simulink model "Modelling"  (R2024b)
settings: Solver=ode15s  StartTime=0.0  StopTime=3*T0  RelTol=1e-7  AbsTol=1e-7
values from neighbouring files (symbols this model uses):
  omega0 = 0    [Numerical_model_1.m]    (also in Numerical_model_2.m = params.omega0)
  omegas = params.omegas    [Numerical_model_2.m]
undefined symbols (not defined in the file or in its folder): params
libraries: fl_lib x26, nesl_utility x12, ee_lib x1
settings Model: Creator=Mihnea  LastModifiedBy=Mihnea
settings SolverCC: AutoScaleAbsTol=off  SolverResetMethod=Robust
settings SimscapeCC: SimscapeLogType=all

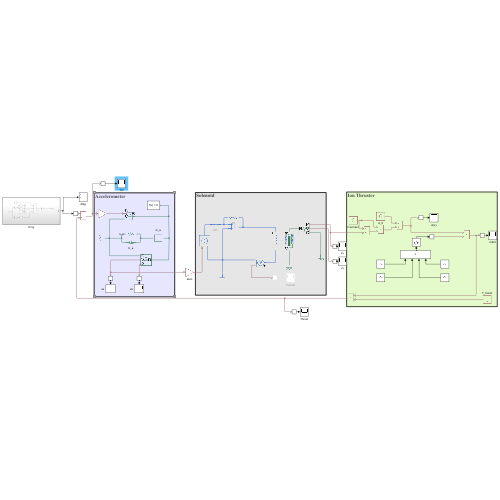
[thumbnail: Simulink's stored preview of the top-level diagram]
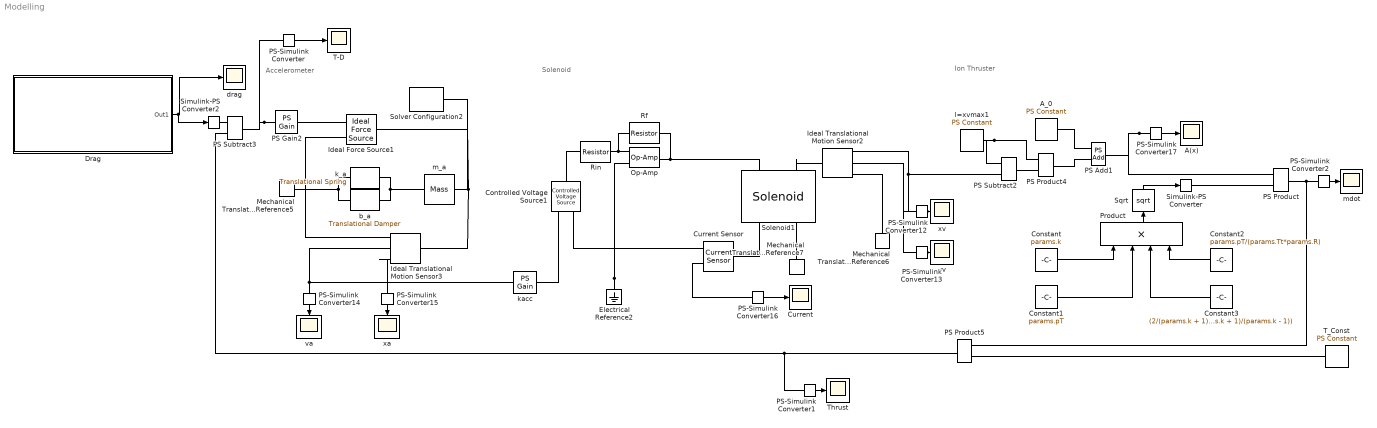
== system Modelling ==
  note: Ion Thruster
  note: Solenoid
  note: Accelerometer
  A(x) : Scope
  A_0 : fl_lib/Physical Signals/Sources/PS Constant  constant=params.A0 m^2
  Constant : Constant  Value=params.k
  Constant1 : Constant  Value=params.pT
  Constant2 : Constant  Value=params.pT/(params.Tt*params.R)
  Constant3 : Constant  Value=(2/(params.k + 1))^((params.k + 1)/(params.k - 1))
  Controlled Voltage Source1 : fl_lib/Electrical/Electrical Sources/Controlled Voltage Source
  Current : Scope
  Current Sensor : fl_lib/Electrical/Electrical Sensors/Current Sensor
  Drag : Subsystem
  Electrical Reference2 : fl_lib/Electrical/Electrical Elements/Electrical Reference
  Ideal Force Source1 : fl_lib/Mechanical/Mechanical Sources/Ideal Force Source
  Ideal Translational Motion Sensor2 : fl_lib/Mechanical/Mechanical Sensors/Ideal Translational Motion Sensor  reference=foundation.enum.MeasurementReference.difference  acceleration_port=false  velocity_port=true  position_port=true  offset=0 m
  Ideal Translational Motion Sensor3 : fl_lib/Mechanical/Mechanical Sensors/Ideal Translational Motion Sensor  reference=foundation.enum.MeasurementReference.difference  acceleration_port=false  velocity_port=true  position_port=true  offset=0 m
  Mechanical Translational Reference5 : fl_lib/Mechanical/Translational Elements/Mechanical Translational Reference
  Mechanical Translational Reference6 : fl_lib/Mechanical/Translational Elements/Mechanical Translational Reference
  Mechanical Translational Reference7 : fl_lib/Mechanical/Translational Elements/Mechanical Translational Reference
  Op-Amp : fl_lib/Electrical/Electrical Elements/Op-Amp  outI_specify=off  outI_priority=None  outI=0 A  outI_nominal_specify=off  outI_nominal_value=1  outI_nominal_unit=A
  PS Add1 : fl_lib/Physical Signals/Functions/PS Add
  PS Gain2 : fl_lib/Physical Signals/Functions/PS Gain  gain=params.ma/params.Msc
  PS Product : fl_lib/Physical Signals/Functions/PS Product
  PS Product4 : fl_lib/Physical Signals/Functions/PS Product
  PS Product5 : fl_lib/Physical Signals/Functions/PS Product
  PS Subtract2 : fl_lib/Physical Signals/Functions/PS Subtract
  PS Subtract3 : fl_lib/Physical Signals/Functions/PS Subtract
  PS-Simulink Converter{,1..2,12..17} (9 alike) : nesl_utility/PS-Simulink Converter  PhysicalDomain=network_engine_domain  SubClassName=ps_output  LeftPortType=input  RightPortType=output  PseudoPeriodic=off  Frequencies=[]  VectorFormat=inherit  Unit=inherit  AffineConversion=off
  Product : Product  Inputs=4
  Rf : fl_lib/Electrical/Electrical Elements/Resistor  R=params.Rf Ohm  i_specify=off  i_priority=None  i=0 A  i_nominal_specify=off  i_nominal_value=1  i_nominal_unit=A  v_specify=off  v_priority=None  v=0 V  v_nominal_specify=off  v_nominal_value=1  v_nominal_unit=V
  Rin : fl_lib/Electrical/Electrical Elements/Resistor  R=params.Rin Ohm  i_specify=off  i_priority=None  i=0 A  i_nominal_specify=off  i_nominal_value=1  i_nominal_unit=A  v_specify=off  v_priority=None  v=0 V  v_nominal_specify=off  v_nominal_value=1  v_nominal_unit=V
  Simulink-PS Converter : nesl_utility/Simulink-PS Converter  PhysicalDomain=network_engine_domain  SubClassName=ps_input  LeftPortType=input  RightPortType=output  PseudoPeriodic=off  Frequencies=[]  NoiseDistribution=none  NoiseParameters=[]  Unit=kg/m^2/s  AffineConversion=off  FilteringAndDerivatives=provide  SimscapeFilterOrder=1  InputFilterTimeConstant=0.001  UdotUserProvided=0
  Simulink-PS Converter2 : nesl_utility/Simulink-PS Converter  PhysicalDomain=network_engine_domain  SubClassName=ps_input  LeftPortType=input  RightPortType=output  PseudoPeriodic=off  Frequencies=[]  NoiseDistribution=none  NoiseParameters=[]  Unit=N  AffineConversion=off  FilteringAndDerivatives=provide  SimscapeFilterOrder=1  InputFilterTimeConstant=0.001  UdotUserProvided=0
  Solenoid1 : ee_lib/Electromechanical/Mechatronic Actuators/Solenoid  motionDirection=ee.enum.actuators.solenoidDirection.away  F12=[9000, 12] N  X12=[0, 0.1] mm  Vdc=0.6 mV  Imax=0.1 A  K=1000 N/m  Xzero=0 mm  lam=1000 N*s/m  Mass=0.1 kg  Xmax=0.1 mm  K_endstop=0.12*1e6 N/m  D_endstop=1e4 N*s/m  i_specify=on  i_priority=High  i=1e-6 A  i_nominal_specify=off  i_nominal_value=-10e-6  i_nominal_unit=A  x_specify=on  x_priority=High  x=1e-6 m  x_nominal_specify=off  x_nominal_value=1  x_nominal_unit=mm  vel_specify=off  vel_priority=High  vel=0.01 mm/s  vel_nominal_specify=off  vel_nominal_value=1  vel_nominal_unit=mm/s  F_specify=off  F_priority=None  F=0 N  F_nominal_specify=off  F_nominal_value=1  F_nominal_unit=N  v_L_specify=off  v_L_priority=None  v_L=0 V  v_L_nominal_specify=off  v_L_nominal_value=1  v_L_nominal_unit=V  magnetic_force_specify=off  magnetic_force_priority=None  magnetic_force=0 N  magnetic_force_nominal_specify=off  magnetic_force_nominal_value=1  magnetic_force_nominal_unit=N  alpha=3.93e-3 1/K  Tmeas=25 degC  thermal_mass=100 J/K  temperature_specify=off  temperature_priority=High  temperature=25 degC  temperature_nominal_specify=off  temperature_nominal_value=1  temperature_nominal_unit=degC  Q_specify=off  Q_priority=None  Q=0 W  Q_nominal_specify=off  Q_nominal_value=1  Q_nominal_unit=W
      settings: InternalSimscapePortConfiguration="{\"Bottom\":[],\"Left\":[{\"id\":\"p\",\"label\":\"+\",\"type\":\"foundation.electrical.electrical\"},{\"id\":\"R\",\"label\":\"R\",\"type\":\"foundation.mechanical.translational.translational\"}],\"Right\":[{\"id\":\"n\",\"label\":\"-\",\"type\":\"foundation.electrical.electrical\"},{\"id\":\"C\",\"label\":\"C\",\"type\":\"foundation.mechanical.translational.translational\"}],\"Top\":[]}"
  Solver Configuration2 : nesl_utility/Solver Configuration  PhysicalDomain=network_engine_domain  SubClassName=solver  LeftPortType=input  RightPortType=generic  Tones=[]  Harmonics=[]  SimulateNoise=off  Profile=off  UseLocalSampling=off  EnableSwitchedLinearOptims=on  FrequencyDomain=off  UseCCode=off  RelTol=0.001  AbsTol=0.001  MinStep=1e-09  ToWorkspace=off  RevertToSquareIcSolve=off  NumHomotopyIterations=100  PhasorMode=off  PhasorModeNumHarmonics=1  ConsistencySolver=NEWTON_XTOL_AFTER_FTOL  IndexReductionMethod=DerivativeReplacement  DoDC=off  ResidualTolerance=1e-09  ConsistencyTolSource=GLOBAL  ConsistencyAbsTol=0.001  ConsistencyRelTol=0.001  ConsistencyTolFactor=1e-6  UseLocalSolver=off  LocalSolverChoice=NE_BACKWARD_EULER_ADVANCER  ResolveIndetEquations=on  FunctionEvalNumThread=1  LocalSolverSampleTime=0.001  DoFixedCost=off  MaxNonlinIter=3  MaxModeIter=2  ComputeImpulses=off  ImpulseIterations=2  LinearAlgebra=auto  LinearAlgebraNumThread=0  EquationFormulation=NE_TIME_EF  DelaysMemoryBudget=1024  AutomaticFiltering=on  FilteringTimeConstant=0.001  PartitionStorageMethod=AS_NEEDED  PartitionMemoryBudget=1024  PartitionMethod=ROBUST  MultibodyUseLocalSolver=on  MultibodyLocalSolverChoice=ODE1  MultibodyLocalSolverSampleTime=0.001
  Sqrt : Sqrt
  T-D : Scope
  T_Const : fl_lib/Physical Signals/Sources/PS Constant  constant=params.Tconst m/s
  Thrust : Scope
  b_a : fl_lib/Mechanical/Translational Elements/Translational Damper  D=params.ba N*s/m  v_specify=on  v_priority=None  v=10^-6 m/s  v_nominal_specify=off  v_nominal_value=1  v_nominal_unit=m/s  f_specify=off  f_priority=None  f=0 N  f_nominal_specify=off  f_nominal_value=1  f_nominal_unit=N
  drag : Scope
  k_a : fl_lib/Mechanical/Translational Elements/Translational Spring  spr_rate=params.ka N/m  v_specify=on  v_priority=None  v=10^-6 m/s  v_nominal_specify=off  v_nominal_value=1  v_nominal_unit=m/s  f_specify=off  f_priority=None  f=0 N  f_nominal_specify=off  f_nominal_value=1  f_nominal_unit=N  x_specify=on  x_priority=High  x=10^-6 m  x_nominal_specify=off  x_nominal_value=1  x_nominal_unit=m
  kacc : fl_lib/Physical Signals/Functions/PS Gain  gain=1 V*s/m
  l=xvmax1 : fl_lib/Physical Signals/Sources/PS Constant  constant=params.xvmax m
  m_a : fl_lib/Mechanical/Translational Elements/Mass  mass=ma kg  num_ports=foundation.enum.numPorts2.two  v_specify=on  v_priority=High  v=10^-6 m/s  v_nominal_specify=off  v_nominal_value=1  v_nominal_unit=m/s  f_specify=off  f_priority=None  f=0 N  f_nominal_specify=off  f_nominal_value=1  f_nominal_unit=N
      settings: InternalSimscapePortConfiguration="{\"Bottom\":[],\"Left\":[{\"id\":\"M\",\"label\":\"\",\"type\":\"foundation.mechanical.translational.translational\"}],\"Right\":[{\"id\":\"N\",\"label\":\"\",\"type\":\"foundation.mechanical.translational.translational\"}],\"Top\":[]}"
  mdot : Scope
  va : Scope
  vv : Scope
  xa : Scope
  xv : Scope
  wires:
  PS-Simulink Converter12/1 -> xv/1
  PS-Simulink Converter13/1 -> vv/1
  PS-Simulink Converter16/1 -> Current/1
  Drag/1(Out1) -> Simulink-PS Converter2/1, drag/1
  PS-Simulink Converter/1 -> T-D/1
  PS-Simulink Converter14/1 -> va/1
  PS-Simulink Converter1/1 -> Thrust/1
  PS-Simulink Converter15/1 -> xa/1
  PS-Simulink Converter17/1 -> A(x)/1
  PS-Simulink Converter2/1 -> mdot/1
  Constant/1 -> Product/1
  Constant1/1 -> Product/2
  Constant2/1 -> Product/4
  Constant3/1 -> Product/3
  Product/1 -> Sqrt/1
  Sqrt/1 -> Simulink-PS Converter/1
  connections:
  Rf/RConn1 -- Solenoid1/LConn1 -- Op-Amp/RConn1
  PS Subtract2/LConn2 -- Ideal Translational Motion Sensor2/RConn3 -- PS-Simulink Converter12/LConn1
  Electrical Reference2/LConn1 -- Op-Amp/LConn1 -- Current Sensor/RConn2 -- Controlled Voltage Source1/RConn2
  PS-Simulink Converter17/LConn1 -- PS Product/LConn1 -- PS Add1/RConn1
  k_a/RConn1 -- Ideal Translational Motion Sensor3/RConn1 -- Ideal Force Source1/RConn2 -- Mechanical Translational Reference5/LConn1 -- b_a/RConn1
  PS Gain2/LConn1 -- PS Subtract3/RConn1 -- PS-Simulink Converter/LConn1
  PS Product5/RConn1 -- PS-Simulink Converter1/LConn1 -- PS Subtract3/LConn1
  b_a/LConn1 -- k_a/LConn1 -- m_a/LConn1
  PS-Simulink Converter14/LConn1 -- kacc/LConn1 -- Ideal Translational Motion Sensor3/RConn2
  Rf/LConn1 -- Rin/RConn1 -- Op-Amp/LConn2
  l=xvmax1/RConn1 -- PS Subtract2/LConn1 -- PS Product4/LConn1
  Ideal Translational Motion Sensor3/RConn3 -- PS-Simulink Converter15/LConn1
  PS-Simulink Converter16/LConn1 -- Current Sensor/RConn1
  Ideal Translational Motion Sensor2/RConn1 -- Mechanical Translational Reference6/LConn1
  Rin/LConn1 -- Controlled Voltage Source1/LConn1
  PS Product5/LConn1 -- T_Const/RConn1
  PS Subtract3/LConn2 -- Simulink-PS Converter2/RConn1
  PS Subtract2/RConn1 -- PS Product4/LConn2
  A_0/RConn1 -- PS Add1/LConn1
  Solenoid1/LConn2 -- Ideal Translational Motion Sensor2/LConn1
  Solenoid1/RConn2 -- Mechanical Translational Reference7/LConn1
  PS Gain2/RConn1 -- Ideal Force Source1/RConn1
  Controlled Voltage Source1/RConn1 -- kacc/RConn1
  PS Product4/RConn1 -- PS Add1/LConn2
  Solenoid1/RConn1 -- Current Sensor/LConn1
  PS-Simulink Converter13/LConn1 -- Ideal Translational Motion Sensor2/RConn2
  m_a/RConn1 -- Ideal Force Source1/LConn1 -- Solver Configuration2/RConn1 -- Ideal Translational Motion Sensor3/LConn1
  PS Product/RConn1 -- PS-Simulink Converter2/LConn1 -- PS Product5/LConn2
  Simulink-PS Converter/RConn1 -- PS Product/LConn2

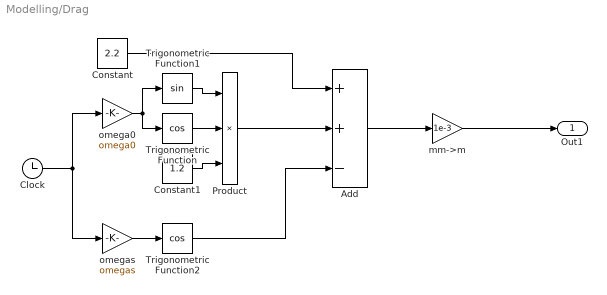
== system Modelling/Drag ==
  Add : Sum  Inputs=++-
  Clock : Clock
  Constant : Constant  Value=2.2
  Constant1 : Constant  Value=1.2
  Product : Product  Inputs=3
  Trigonometric Function : Trigonometry  Operator=cos
  Trigonometric Function1 : Trigonometry
  Trigonometric Function2 : Trigonometry  Operator=cos
  mm->m : Gain  Gain=1e-3
  omega0 : Gain  Gain=omega0
  omegas : Gain  Gain=omegas
  Out1 : Outport
  wires:
  Clock/1 -> omega0/1, omegas/1
  Trigonometric Function1/1 -> Product/1
  Trigonometric Function/1 -> Product/2
  Constant1/1 -> Product/3
  omega0/1 -> Trigonometric Function1/1, Trigonometric Function/1
  Constant/1 -> Add/1
  Product/1 -> Add/2
  Trigonometric Function2/1 -> Add/3
  omegas/1 -> Trigonometric Function2/1
  Add/1 -> mm->m/1
  mm->m/1 -> Out1/1
